simulink model "SI_test"  (R2022a)
settings: Solver=ode4  StartTime=0.0  StopTime=300  FixedStep=1e-5  RelTol=1e-3  AbsTol=1e-3
libraries: spspowerguiLib x1
settings Model: Creator=ujjwo  LastModifiedBy=niran
settings SolverCC: AutoScaleAbsTol=off  AlgebraicLoopSolver=TrustRegion  AutoInsertRateTranBlk=on
settings DataIOCC: LimitDataPoints=on  MaxDataPoints=10000  ReturnWorkspaceOutputs=off
settings OptimizationCC: EfficientMapNaN2IntZero=off  LifeSpan=inf
settings DebuggingCC: AllowSymbolicDim=off  SFUnexpectedBacktrackingDiag=warning  SFNoUnconditionalDefaultTransitionDiag=warning  SFExecutionAtInitializationDiag=none  SFMachineParentedDataDiag=warning  ArithmeticOperatorsInVariantConditions=warning
settings HardwareCC: TargetBitPerPointer=64  TargetBitPerSizeT=64  TargetBitPerPtrDiffT=64  TargetLongLongMode=on  TargetIntDivRoundTo=Zero  TargetEndianess=LittleEndian  TargetWordSize=64  TargetHWDeviceType=MATLAB Host  ProdEqTarget=off
settings SFSimCC: SimUseLocalCustomCode=off  CustomCodeUndefinedFunction=UseInterfaceOnly
settings RTWCC: GenCodeOnly=on  PackageGeneratedCodeAndArtifacts=on  PackageName=TestResult.zip
settings CodeAppCC: MaxIdLength=128
settings GRTTargetCC: TargetLangStandard=C89/C90 (ANSI)  GenerateFullHeader=off  CombineOutputUpdateFcns=off  MatFileLogging=off
settings ConfigComp: CovMetricSettings=dw  CovSaveCumulativeToWorkspaceVar=on  CovSaveSingleToWorkspaceVar=on  CovExternalEMLEnable=off  CovSFcnEnable=off
settings SimscapeCC: SimscapeLogType=all  SimscapeLogDataHistory=10000

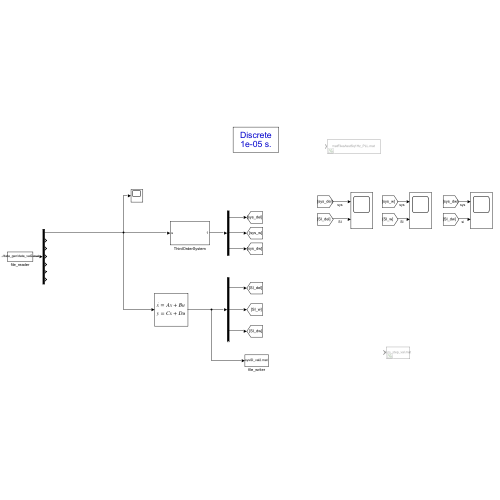
[thumbnail: Simulink's stored preview of the top-level diagram]
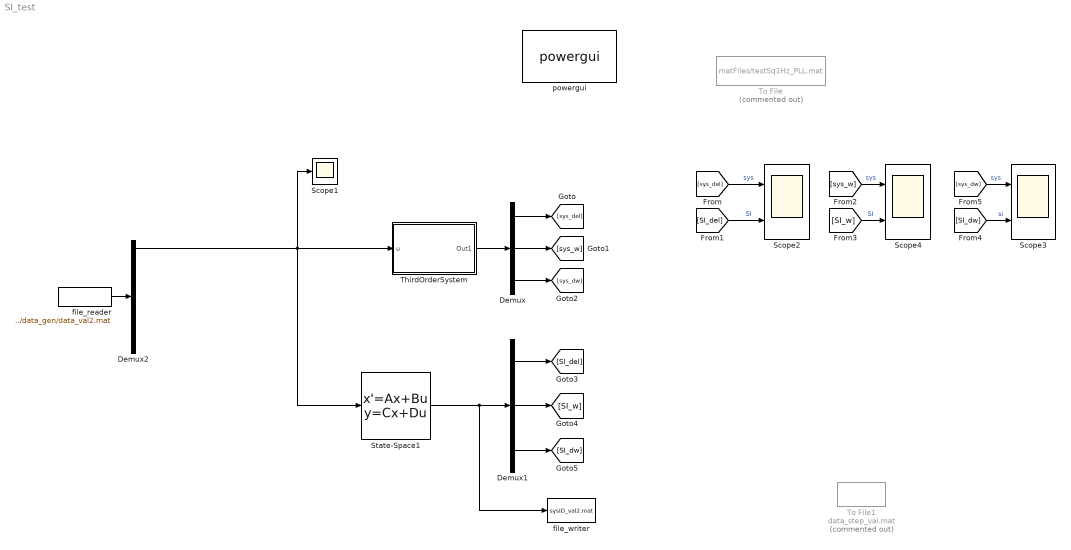
== system SI_test ==
  Demux : Demux  Outputs=3
  Demux1 : Demux  Outputs=3
  Demux2 : Demux  Outputs=7
  Scope1 : Scope
  Scope2 : Scope  NumInputPorts=2
  Scope3 : Scope  NumInputPorts=2
  Scope4 : Scope  NumInputPorts=2
  State-Space1 : StateSpace  A=|  B=|  C=eye(3)  D=[0;0;0]  InitialCondition=0
      A=|
      | [0, 1.0, 0;
      | 0, 0, 1;
      | -2.0700425260532183, -26.739610499177303, -5.351435222623707]
      B=|
      | [-0.009099383338581388;
      | -0.000870938932030332;
      | -1.24145686633005]
  ThirdOrderSystem : Subsystem
  To File : ToFile  Commented=on  Filename=matFiles/testSq1Hz_PLL.mat  MatrixName=datavar  SampleTime=0.02
  To File1 : ToFile  Commented=on  Filename=data_step_val.mat  MatrixName=datavar  SampleTime=0.02
  file_reader : FromFile  FileName=../data_gen/data_val2.mat  OutDataTypeStr=double  SampleTime=0
  file_writer : ToFile  Filename=sysID_val2.mat  MatrixName=datavar  SampleTime=0.02
  powergui : spspowerguiLib/powergui  Priority=1  SimulationMode=Discrete  SampleTime=1e-5  frequency=60  Iterations=50  frequencyindice=60  Pbase=100e6  ErrMax=0.0001  UnitsV=kV  UnitsW=MW  buscounter=3  FunctionMessages=off  echomessages=off  EnableUseOfTLC=off  CurrentSourceSwitches=off  DisableSnubberDevices=off  DisableRonSwitches=off  DisableVfSwitches=off  DisplayEquations=off  AutomaticDiscreteSolvers=off  SolverType=Tustin  Interpol=off  ExternalGateDelay=off  methode=off  Ts=100  x0status=steady  SPID=on  SwTol=0  HookPort=off  NonlinearTolerance=1e-4  nMaxIteration=100  ContinueOnMaxIteration=off  RestoreLinks=warning  ResistiveCurrentMeasurement=off  Frange=[0:2:500]  Ylog=off  Xlog=on  ShowGrid=off  save=off  variable=ZData  structure=0  ZoomFFT=off  StartTime=0.0  cycles=1  DisplayStyle=1  fundamental=60  FreqAxis=off  MaxFrequency=1000  frequencyindicesteady=1  RmsSteady=2  display=off
  wires:
  ThirdOrderSystem/1(Out1) -> Demux/1
  Demux/1 -> [sys_del]
  Demux/2 -> [sys_w]
  Demux/3 -> [sys_dw]
  Demux1/1 -> [SI_del]
  Demux1/2 -> [SI_w]
  Demux1/3 -> [SI_dw]
  [sys_del] -> Scope2/1  "sys"
  [SI_del] -> Scope2/2  "SI"
  [sys_w] -> Scope4/1  "sys"
  [SI_w] -> Scope4/2  "SI"
  [SI_dw] -> Scope3/2  "si"
  [sys_dw] -> Scope3/1  "sys"
  Demux2/1 -> State-Space1/1, ThirdOrderSystem/1(u), Scope1/1
  file_reader/1 -> Demux2/1
  State-Space1/1 -> file_writer/1, Demux1/1

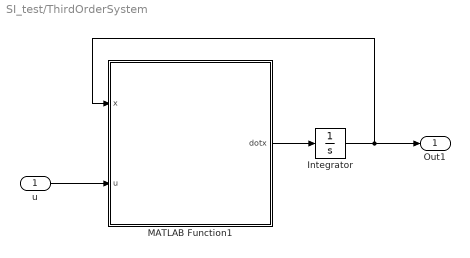
== system SI_test/ThirdOrderSystem ==
  u : Inport
  Integrator : Integrator  InitialCondition=[0;0;0]
  MATLAB Function1 : MATLAB Function  TreatAsAtomicUnit=on
  Out1 : Outport
  wires:
  MATLAB Function1/1(dotx) -> Integrator/1
  Integrator/1 -> Out1/1, MATLAB Function1/1(x)
  u/1 -> MATLAB Function1/2(u)

== matlab function SI_test/ThirdOrderSystem/MATLAB Function1 ==
  data: x input; u input; dotx output
function dotx = ThirdOrderSystem(x, u)
% M = 4; D = 1.5; Rp = 0.05; Tg = 0.2; Ki =1.8;
% A = [ 0, 1; -(D/(M*Tg) + 1/(Rp*M*Tg)), -(D/M+1/Tg)];
% B = [0; (1/(M*Tg))];
% dotx = A*x + B*u;
    ki = 2;
    Tg = 0.2;
    Rp = 0.05;
    
    de = x(1);
    w = x(2);
    wdot= x(3);

    M = 4.0;
    D = 1.5;

    dotx =  [
        w;
        wdot;
        -(ki/(M*Tg))*de-(D/(M*Tg) + 1/(Rp*M*Tg))*w - (D/M+1/Tg)*wdot - 1/(M*Tg) * u
    ];
